simulink model "Cruise_Control"  (R2020b)
settings: Solver=VariableStepAuto  StartTime=0.0  StopTime=120.0  RelTol=1e-3
values from neighbouring files (symbols this model uses):
  b = 50.0    [Problem3.sldd]
  m = 1000.0    [Problem3.sldd]
settings Model: DataDictionary=Problem3.sldd  Creator=Shirish  LastModifiedBy=Shirish
settings DataIOCC: SaveOutput=off  SaveTime=off

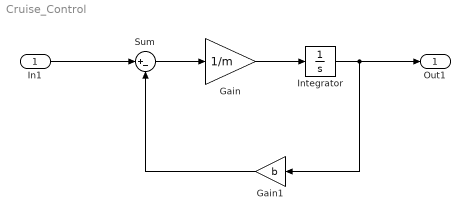
== system Cruise_Control ==
  In1 : Inport  OutDataTypeStr=double  PortDimensions=1  SampleTime=0
  Gain : Gain  Gain=1/m
  Gain1 : Gain  Gain=b
  Integrator : Integrator
  Sum : Sum  Inputs=|+-
  Out1 : Outport  OutDataTypeStr=double  PortDimensions=1  SampleTime=0
  wires:
  Integrator/1 -> Gain1/1, Out1/1
  Sum/1 -> Gain/1
  Gain/1 -> Integrator/1
  Gain1/1 -> Sum/2
  In1/1 -> Sum/1
